simulink model "ESTS_VGMG_test"  (R2023b)
settings: Solver=VariableStepAuto  StartTime=0.0  StopTime=10.0  RelTol=1e-3
libraries: simulink x1, ESTS_VGMG x1
settings Model: Creator=blatak  LastModifiedBy=blatak

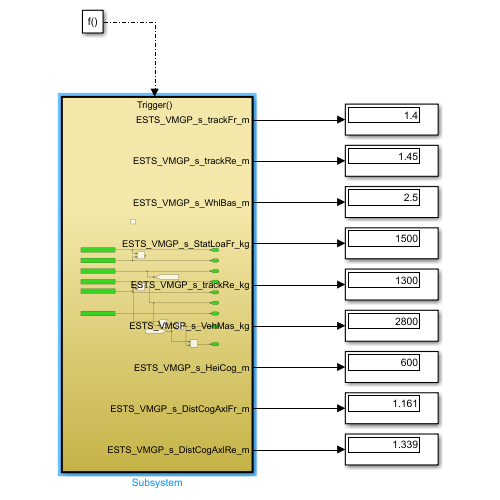
[thumbnail: Simulink's stored preview of the top-level diagram]
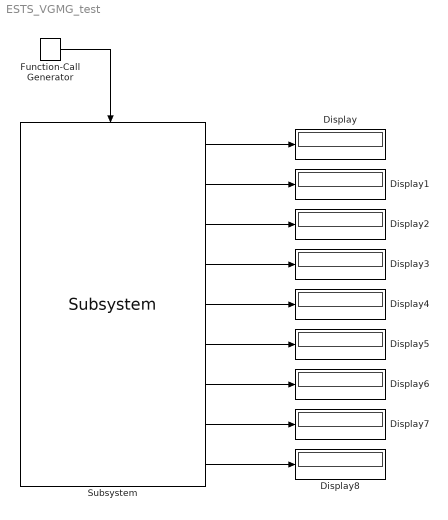
== system ESTS_VGMG_test ==
  Display{,1..8} (9 alike) : Display
  Function-Call Generator : simulink/Ports & Subsystems/Function-Call Generator  sample_time=0.01  numberOfIterations=1  DisallowWideOutput=off
  Subsystem : ESTS_VGMG/Subsystem  SystemSampleTime=-1  VariantActivationTime=update diagram  AllowFlexibleInterface=on  Latency=0  AutoFrameSizeCalculation=off
  wires:
  Function-Call Generator/1 -> Subsystem/Trigger
  Subsystem/1 -> Display/1
  Subsystem/2 -> Display1/1
  Subsystem/3 -> Display2/1
  Subsystem/4 -> Display3/1
  Subsystem/5 -> Display4/1
  Subsystem/6 -> Display5/1
  Subsystem/7 -> Display6/1
  Subsystem/8 -> Display7/1
  Subsystem/9 -> Display8/1
